simulink model "diodevmax180v"  (R2018a)
settings: Solver=VariableStepAuto  StartTime=0.0  StopTime=1  RelTol=1e-3
libraries: powerlib x18
settings Model: Creator=c  LastModifiedBy=c

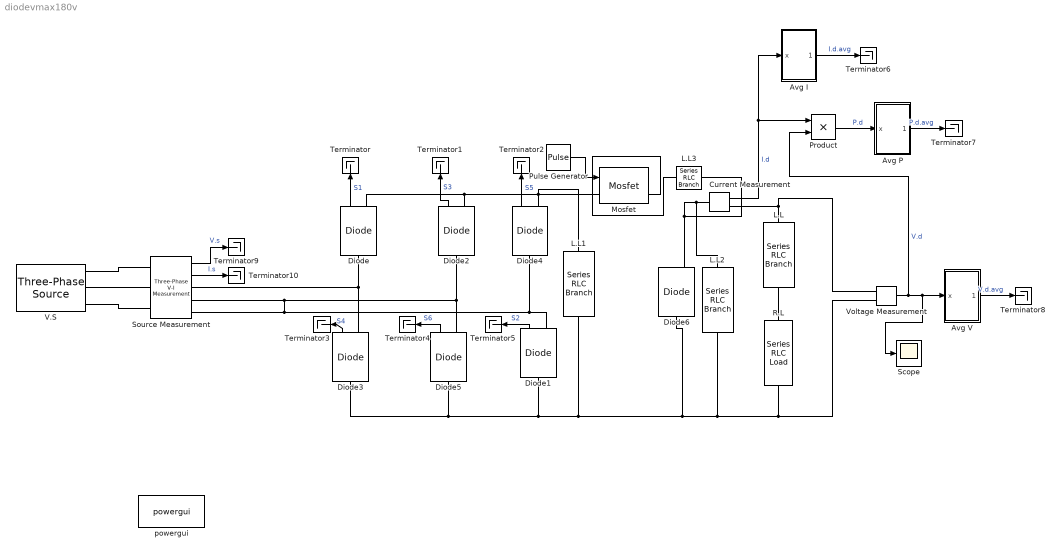
== system diodevmax180v ==
  Avg I : Subsystem
  Avg P : Subsystem
  Avg V : Subsystem
  Current Measurement : powerlib/Measurements/Current Measurement  PhasorSimulation=off  OutputType=Complex  PSBequivalent=0
  Diode{,1..6} (7 alike) : powerlib/Power Electronics/Diode  Ron=0.001  Lon=0  Vf=0.8  IC=0  UseSnubber=0  Rs=500  Cs=250e-9  Measurements=on
  L.L : powerlib/Elements/Series RLC Branch  LConnTagsString=__new0  RConnTagsString=__new0  BranchType=L  Resistance=1  Inductance=1e-5  SetiL0=off  InitialCurrent=0  Capacitance=1e-6  Setx0=off  InitialVoltage=0  Measurements=None
  L.L1 : powerlib/Elements/Series RLC Branch  LConnTagsString=__new0  RConnTagsString=__new0  BranchType=C  Resistance=1  Inductance=1e-5  SetiL0=off  InitialCurrent=0  Capacitance=1e-3  Setx0=off  InitialVoltage=0  Measurements=None
  L.L2 : powerlib/Elements/Series RLC Branch  LConnTagsString=__new0  RConnTagsString=__new0  BranchType=C  Resistance=1  Inductance=1e-5  SetiL0=off  InitialCurrent=0  Capacitance=200e-6  Setx0=off  InitialVoltage=0  Measurements=None
  L.L3 : powerlib/Elements/Series RLC Branch  LConnTagsString=__new0  RConnTagsString=__new0  BranchType=L  Resistance=1  Inductance=10e-5  SetiL0=off  InitialCurrent=0  Capacitance=1e-6  Setx0=off  InitialVoltage=0  Measurements=None
  Mosfet : powerlib/Power Electronics/Mosfet  Ron=0.1  Lon=0  Rd=0.01  Vfd=0  IC=0  Rs=1e5  Cs=inf  Measurements=on
  Product : Product
  Pulse Generator : DiscretePulseGenerator  PulseType=Time based  Period=1/10000  PulseWidth=20
  R.L : powerlib/Elements/Series RLC Load  LConnTagsString=a  RConnTagsString=__new0  NominalVoltage=220  NominalFrequency=50  ActivePower=1.6e3  InductivePower=0  CapacitivePower=0  Setx0=off  InitialVoltage=0  SetiL0=off  InitialCurrent=0  Measurements=None  LoadType=constant Z
  Scope : Scope
  Source Measurement : powerlib/Measurements/Three-Phase V-I Measurement  VoltageMeasurement=phase-to-ground  SetLabelV=off  LabelV=Vabc  Vpu=off  VpuLL=off  CurrentMeasurement=yes  SetLabelI=off  LabelI=Iabc  Ipu=off  Pbase=100e6  Vbase=500e3  OutputType=Complex  PhasorSimulation=off  PSBequivalent=0
  Terminator{,1..10} (11 alike) : Terminator
  V.S : powerlib/Electrical Sources/Three-Phase Source  InternalConnection=Yg  VoltagePhases=off  Voltage=220*sqrt(3)  PhaseAngle=0  Voltage_phases=[25e3 25e3 25e3]/sqrt(3)  PhaseAngles_phases=[0 -120 +120]  Frequency=50  NonIdealSource=on  SpecifyImpedance=on  Resistance=0.8929  Inductance=16.58e-3  ShortCircuitLevel=sqrt(3)*220*20000  BaseVoltage=220*sqrt(3)  XRratio=0.1  BusType=swing  Pref=10e3  Qref=0  Prefabc=[10e3, 10e3, 10e3]  Qrefabc=[0, 0, 0]  Qmin=-inf  Qmax=inf
  Voltage Measurement : powerlib/Measurements/Voltage Measurement  PhasorSimulation=off  OutputType=Complex  PSBequivalent=0
  powergui : powerlib/powergui  Priority=1  SimulationMode=Continuous  SampleTime=50e-6  frequency=60  Iterations=50  frequencyindice=0  Pbase=100e6  ErrMax=1e-4  UnitsV=kV  UnitsW=MW  buscounter=0  FunctionMessages=off  echomessages=off  EnableUseOfTLC=off  CurrentSourceSwitches=off  DisableSnubberDevices=off  DisableRonSwitches=off  DisableVfSwitches=off  DisplayEquations=off  SolverType=Tustin/Backward Euler (TBE)  Interpol=off  ExternalGateDelay=off  methode=off  Ts=100  x0status=blocks  SPID=on  SwTol=0  HookPort=off  RestoreLinks=warning  ResistiveCurrentMeasurement=off  Frange=[0:2:500]  Ylog=off  Xlog=on  ShowGrid=off  save=off  variable=ZData  structure=0  ZoomFFT=off  StartTime=0.0  cycles=1  DisplayStyle=1  fundamental=60  FreqAxis=off  MaxFrequency=1000  frequencyindicesteady=1  RmsSteady=1  display=off
  wires:
  Avg V/1(x.avg) -> Terminator8/1  "V.d.avg"
  Diode5/1 -> Terminator4/1  "S6"
  Diode4/1 -> Terminator2/1  "S5"
  Diode3/1 -> Terminator3/1  "S4"
  Voltage Measurement/1 -> Scope/1, Avg V/1(x), Product/2  "V.d"
  Diode/1 -> Terminator/1  "S1"
  Diode1/1 -> Terminator5/1  "S2"
  Source Measurement/1 -> Terminator9/1  "V.s"
  Diode2/1 -> Terminator1/1  "S3"
  Current Measurement/1 -> Avg I/1(x), Product/1  "I.d"
  Avg I/1(x.avg) -> Terminator6/1  "I.d.avg"
  Source Measurement/2 -> Terminator10/1  "I.s"
  Product/1 -> Avg P/1(x)  "P.d"
  Avg P/1(x.avg) -> Terminator7/1  "P.d.avg"
  Pulse Generator/1 -> Mosfet/1
  connections:
  Diode/RConn1 -- L.L1/LConn1 -- Mosfet/LConn1 -- Diode4/RConn1 -- Diode2/RConn1
  L.L/LConn1 -- Current Measurement/RConn1 -- Voltage Measurement/LConn1
  Source Measurement/RConn1 -- Diode/LConn1 -- Diode3/RConn1
  Source Measurement/RConn2 -- Diode1/RConn1 -- Diode4/LConn1 -- Source Measurement/RConn3 -- Diode5/RConn1 -- Diode2/LConn1
  V.S/RConn3 -- Source Measurement/LConn3
  V.S/RConn2 -- Source Measurement/LConn2
  L.L/RConn1 -- R.L/LConn1
  V.S/RConn1 -- Source Measurement/LConn1
  Diode1/LConn1 -- Diode6/LConn1 -- L.L2/RConn1 -- Voltage Measurement/LConn2 -- R.L/RConn1 -- L.L1/RConn1 -- Diode5/LConn1 -- Diode3/LConn1
  Diode6/RConn1 -- L.L2/LConn1 -- Current Measurement/LConn1 -- L.L3/LConn1
  Mosfet/RConn1 -- L.L3/RConn1

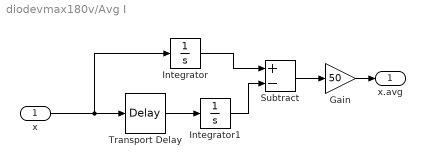
== system diodevmax180v/Avg I ==
  x : Inport
  Gain : Gain  Gain=50
  Integrator : Integrator
  Integrator1 : Integrator
  Subtract : Sum  Inputs=+-
  Transport Delay : TransportDelay  DelayTime=1/50
  x.avg : Outport
  wires:
  Transport Delay/1 -> Integrator1/1
  Integrator/1 -> Subtract/1
  Integrator1/1 -> Subtract/2
  x/1 -> Integrator/1, Transport Delay/1
  Gain/1 -> x.avg/1
  Subtract/1 -> Gain/1

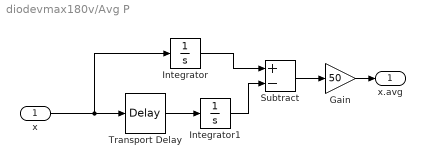
== system diodevmax180v/Avg P ==
  x : Inport
  Gain : Gain  Gain=50
  Integrator : Integrator
  Integrator1 : Integrator
  Subtract : Sum  Inputs=+-
  Transport Delay : TransportDelay  DelayTime=1/50
  x.avg : Outport
  wires:
  Transport Delay/1 -> Integrator1/1
  Integrator/1 -> Subtract/1
  Integrator1/1 -> Subtract/2
  x/1 -> Integrator/1, Transport Delay/1
  Gain/1 -> x.avg/1
  Subtract/1 -> Gain/1

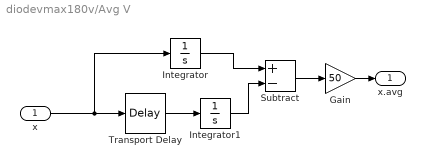
== system diodevmax180v/Avg V ==
  x : Inport
  Gain : Gain  Gain=50
  Integrator : Integrator
  Integrator1 : Integrator
  Subtract : Sum  Inputs=+-
  Transport Delay : TransportDelay  DelayTime=1/50
  x.avg : Outport
  wires:
  Transport Delay/1 -> Integrator1/1
  Integrator/1 -> Subtract/1
  Integrator1/1 -> Subtract/2
  x/1 -> Integrator/1, Transport Delay/1
  Gain/1 -> x.avg/1
  Subtract/1 -> Gain/1
